simulink model "Model_IPS7"  (R2016a)
settings: Solver=FixedStepAuto  StartTime=0  StopTime=560  FixedStep=1e-5
InitFcn:
  | parametriAM
values from neighbouring files (symbols this model uses):
  Imrn = 7.4    [parametriAM.m]
  Ismax = In*sqrt(2)    [parametriAM.m]
  J = 0.019    [parametriAM.m]    (also in podatki.m = 0.01)
  Ki_Imr = 1000    [parametriAM.m]
  Ki_tok = 5.0    (= 5)    [parametriAM.m]
  Ki_wr = 1000    [parametriAM.m]
  Kp_Imr = 100    [parametriAM.m]
  Kp_tok = 0.05    [parametriAM.m]
  Kp_wr = 50    [parametriAM.m]
  Lm = 0.0493    [parametriAM.m]    (also in podatki.m = 0.2342)
  Lr = 0.05315    [parametriAM.m]    (also in podatki.m = 0.2449)
  Ls = 0.05315    [parametriAM.m]    (also in podatki.m = 0.2449)
  Lst = sigma*Ls    (= 0.00742111947319)    [parametriAM.m]
  naklon = naklon    [parametriAM.m]    (also in staticna_karakteristika.m = 1.0471975512)
  pp = 3    [parametriAM.m]    (also in podatki.m = 2)
  Rs = 0.594    [parametriAM.m]    (also in podatki.m = 3.7)
  sigma = 1 - 1/((1+sigmaR)*(1+sigmaS))    (= 0.13962595434)    [parametriAM.m]
  static_or_dinamic = static_or_dinamic    [parametriAM.m]    (also in potek_toka.m = 0; staticna_karakteristika.m = 5)
  Tr = Lr/Rr    (= 0.0771407837446)    [parametriAM.m]
  Udc = Un*sqrt(2)    [parametriAM.m]
  wb_upper_limit_field_weaking = sqrt((Ls^2+Lst^2)/(2*Lst^2*Ls^2))*Usmax/Ismax    [parametriAM.m]
  wdod = 2000*2*pi/60    (= 209.439510239)    [parametriAM.m]
  wn = Udc/sqrt(Ls^2*(Imrn)^2+Lst^2*(Ismax^2-(Imrn)^2))    [maximalnaelipsa.m]    (also in parametriAM.m = Un/sqrt(Ls^2*(Imrn)^2+Lst^2*(Ismax^2-(Imrn)^2))/pp)
libraries: simulink x25
(part 2 of 2)

== system Model_IPS7/Asinhronski stroj2/napetostni dq model/eq 5.46 ==
  Usd : Inport
  dImr/dt : Inport  Port=2
  Isq : Inport  Port=3
  wmr : Inport  Port=4
  Gain : Gain  Gain=1/(sigma*Ls)
  Gain1 : Gain  Gain=Rs
  Gain2 : Gain  Gain=(1-sigma)*Ls
  Gain3 : Gain  Gain=sigma*Ls
  Integrator : Integrator
  Product : Product  RndMeth=Zero
  Sum : Sum  Inputs=+--+
  Isd : Outport
  wires:
  Gain3/1 -> Sum/4
  Product/1 -> Gain3/1
  Isq/1 -> Product/1
  wmr/1 -> Product/2
  Gain2/1 -> Sum/3
  dImr/dt/1 -> Gain2/1
  Gain1/1 -> Sum/2
  Usd/1 -> Sum/1
  Sum/1 -> Gain/1
  Gain/1 -> Integrator/1
  Integrator/1 -> Gain1/1, Isd/1

== system Model_IPS7/Asinhronski stroj2/napetostni dq model/eq 5.47 ==
  Usq : Inport
  Imr : Inport  Port=2
  Isd : Inport  Port=3
  wmr : Inport  Port=4
  Gain : Gain  Gain=1/(sigma*Ls)
  Gain1 : Gain  Gain=Rs
  Gain2 : Gain  Gain=(1-sigma)*Ls
  Gain3 : Gain  Gain=sigma*Ls
  Integrator : Integrator
  Product : Product  RndMeth=Zero
  Product1 : Product  RndMeth=Zero
  Sum : Sum  Inputs=+---
  Isq : Outport
  wires:
  Gain3/1 -> Sum/4
  Product1/1 -> Gain3/1
  Isd/1 -> Product1/2
  Gain2/1 -> Sum/3
  Product/1 -> Gain2/1
  wmr/1 -> Product1/1, Product/2
  Imr/1 -> Product/1
  Gain1/1 -> Sum/2
  Usq/1 -> Sum/1
  Sum/1 -> Gain/1
  Gain/1 -> Integrator/1
  Integrator/1 -> Gain1/1, Isq/1

== system Model_IPS7/Asinhronski stroj3/Clarke/ABC_ab1 ==
  A : Inport
  B : Inport  Port=2
  C : Inport  Port=3
  Gain1 : Gain  Gain=2
  Gain2 : Gain
  Gain24 : Gain  Gain=sqrt(3)/3
  Sum11 : Sum
  Terminator : Terminator
  alfa : Outport
  beta : Outport  Port=2
  wires:
  A/1 -> Gain2/1, Sum11/1
  Sum11/1 -> Gain24/1
  Gain2/1 -> alfa/1
  Gain24/1 -> beta/1
  B/1 -> Gain1/1
  Gain1/1 -> Sum11/2
  C/1 -> Terminator/1

== system Model_IPS7/Asinhronski stroj3/Inverzni Clarke/ab_ABC ==
  alfa : Inport
  beta : Inport  Port=2
  Gain1 : Gain
  Gain2 : Gain  Gain=-0.5
  Gain25 : Gain  Gain=sqrt(3)/2
  Gain3 : Gain  Gain=sqrt(3)/2
  Gain4 : Gain  Gain=0.5
  Sum10 : Sum
  Sum11 : Sum  Inputs=--
  A : Outport
  B : Outport  Port=2
  C : Outport  Port=3
  wires:
  Sum11/1 -> C/1
  Sum10/1 -> B/1
  Gain1/1 -> A/1
  alfa/1 -> Gain4/1, Gain2/1, Gain1/1
  Gain2/1 -> Sum10/1
  Gain25/1 -> Sum10/2
  Gain4/1 -> Sum11/1
  beta/1 -> Gain3/1, Gain25/1
  Gain3/1 -> Sum11/2

== system Model_IPS7/Asinhronski stroj3/Mehanika/eq 2.19 ==
  M : Inport
  Gain1 : Gain  Gain=1/J
  Integrator : Integrator
  wr : Outport
  wires:
  Gain1/1 -> Integrator/1
  M/1 -> Gain1/1
  Integrator/1 -> wr/1

== system Model_IPS7/Asinhronski stroj3/napetostni dq model/eq 5.35 ==
  Imr : Inport
  Isq : Inport  Port=2
  Gain : Gain  Gain=3*pp/2
  Gain2 : Gain  Gain=Lm*Lm/Lr
  Product : Product  RndMeth=Zero
  Mel : Outport
  wires:
  Imr/1 -> Product/1
  Isq/1 -> Product/2
  Product/1 -> Gain/1
  Gain2/1 -> Mel/1
  Gain/1 -> Gain2/1

== system Model_IPS7/Asinhronski stroj3/napetostni dq model/eq 5.39 ==
  Isd : Inport
  Gain : Gain  Gain=1/Tr
  Integrator : Integrator  InitialCondition=1e-3
  Sum : Sum  Inputs=|+-
  Imr : Outport
  dImr/dt : Outport  Port=2
  wires:
  Isd/1 -> Sum/1
  Integrator/1 -> Imr/1, Sum/2
  Sum/1 -> Gain/1
  Gain/1 -> Integrator/1, dImr/dt/1

== system Model_IPS7/Asinhronski stroj3/napetostni dq model/eq 5.40 ==
  Imr : Inport
  Isq : Inport  Port=2
  wr_el : Inport  Port=3
  Divide : Product  Inputs=*/
  Gain2 : Gain  Gain=Tr
  Saturation : Saturate  UpperLimit=2*pi*50  LowerLimit=-2*pi*50
  Sum : Sum  Inputs=|++
  wmr : Outport
  wires:
  Isq/1 -> Divide/1
  Imr/1 -> Gain2/1
  Gain2/1 -> Divide/2
  Divide/1 -> Saturation/1  "ws"
  wr_el/1 -> Sum/2
  Sum/1 -> wmr/1
  Saturation/1 -> Sum/1

== system Model_IPS7/Asinhronski stroj3/napetostni dq model/eq 5.46 ==
  Usd : Inport
  dImr/dt : Inport  Port=2
  Isq : Inport  Port=3
  wmr : Inport  Port=4
  Gain : Gain  Gain=1/(sigma*Ls)
  Gain1 : Gain  Gain=Rs
  Gain2 : Gain  Gain=(1-sigma)*Ls
  Gain3 : Gain  Gain=sigma*Ls
  Integrator : Integrator
  Product : Product  RndMeth=Zero
  Sum : Sum  Inputs=+--+
  Isd : Outport
  wires:
  Integrator/1 -> Isd/1, Gain1/1
  Gain/1 -> Integrator/1
  Sum/1 -> Gain/1
  Usd/1 -> Sum/1
  Gain1/1 -> Sum/2
  dImr/dt/1 -> Gain2/1
  Gain2/1 -> Sum/3
  wmr/1 -> Product/2
  Isq/1 -> Product/1
  Product/1 -> Gain3/1
  Gain3/1 -> Sum/4

== system Model_IPS7/Asinhronski stroj3/napetostni dq model/eq 5.47 ==
  Usq : Inport
  Imr : Inport  Port=2
  Isd : Inport  Port=3
  wmr : Inport  Port=4
  Gain : Gain  Gain=1/(sigma*Ls)
  Gain1 : Gain  Gain=Rs
  Gain2 : Gain  Gain=(1-sigma)*Ls
  Gain3 : Gain  Gain=sigma*Ls
  Integrator : Integrator
  Product : Product  RndMeth=Zero
  Product1 : Product  RndMeth=Zero
  Sum : Sum  Inputs=+---
  Isq : Outport
  wires:
  Integrator/1 -> Isq/1, Gain1/1
  Gain/1 -> Integrator/1
  Sum/1 -> Gain/1
  Usq/1 -> Sum/1
  Gain1/1 -> Sum/2
  Imr/1 -> Product/1
  wmr/1 -> Product/2, Product1/1
  Product/1 -> Gain2/1
  Gain2/1 -> Sum/3
  Isd/1 -> Product1/2
  Product1/1 -> Gain3/1
  Gain3/1 -> Sum/4

== system Model_IPS7/Regulacija1/Regulacija navora/Limita q toka ==
  Iddej : Inport
  wmr : Inport  Port=2
  Iq* : Inport  Port=3
  0 : Constant  Value=0
  Saturation napetost : simulink/Discontinuities/Saturation Dynamic  OutMin=[]  OutMax=[]  OutDataTypeStr=Inherit: Same as second input  OutDataType=fixdt(1, 16)  OutScaling=2^-10  DoSatur=off
  Saturation presek : simulink/Discontinuities/Saturation Dynamic  OutMin=[]  OutMax=[]  OutDataTypeStr=Inherit: Same as second input  OutDataType=fixdt(1, 16)  OutScaling=2^-10  DoSatur=off
  Saturation tok : simulink/Discontinuities/Saturation Dynamic  OutMin=[]  OutMax=[]  OutDataTypeStr=Inherit: Same as second input  OutDataType=fixdt(1, 16)  OutScaling=2^-10  DoSatur=off
  napetostna limita : Subsystem
  tokovna : Subsystem
  Iqmaxlim : Outport
  Iq*_lim : Outport  Port=2
  wires:
  wmr/1 -> napetostna limita/2(w)
  napetostna limita/1(high) -> Saturation napetost/1, Saturation presek/1
  Iddej/1 -> napetostna limita/1(Iddej), tokovna/1(Id)
  tokovna/2(low) -> Saturation tok/3
  tokovna/1(high) -> Saturation tok/1, Saturation presek/2
  Saturation presek/1 -> Iqmaxlim/1
  Saturation tok/1 -> Saturation napetost/2
  Iq*/1 -> Saturation tok/2
  0/1 -> Saturation presek/3
  napetostna limita/2(low) -> Saturation napetost/3
  Saturation napetost/1 -> Iq*_lim/1

== system Model_IPS7/Regulacija1/Regulacija navora/izracun w_mr ==
  Id : Inport
  Iq : Inport  Port=2
  w : Inport  Port=3
  Constant : Constant  Value=0.00001
  Divide : Product  Inputs=/*
  Gain2 : Gain  Gain=Tr
  Saturation1 : Saturate  UpperLimit=2*pi*50  LowerLimit=-2*pi*50
  Sum : Sum  Inputs=|++
  Sum1 : Sum  Inputs=++|
  Transfer Fcn : TransferFcn  Denominator=[Tr 1]
  wmr : Outport
  wires:
  w/1 -> Sum/2
  Id/1 -> Transfer Fcn/1
  Saturation1/1 -> Sum/1
  Sum/1 -> wmr/1
  Iq/1 -> Divide/2
  Transfer Fcn/1 -> Gain2/1
  Divide/1 -> Saturation1/1
  Gain2/1 -> Sum1/2
  Sum1/1 -> Divide/1
  Constant/1 -> Sum1/1

== system Model_IPS7/Regulacija1/Tok regulator/Dregulator ==
  Id* : Inport
  Iddej : Inport  Port=2
  1/Ti : Gain  Gain=Ki_tok  SaturateOnIntegerOverflow=on  OutDataTypeStr=Inherit: Same as input  ParamDataTypeStr=Inherit: Same as input
  Abs : Abs  ZeroCross=off
  Add2 : Sum  Inputs=+-
  Compare To Zero : simulink/Logic and Bit Operations/Compare To Zero  relop=<=  OutDataTypeStr=boolean  ZeroCross=off
  Integrator : Integrator
  Kp : Gain  Gain=Kp_tok  SaturateOnIntegerOverflow=on  OutDataTypeStr=Inherit: Same as input  ParamDataTypeStr=Inherit: Same as input
  Product : Product
  Saturation : Saturate  UpperLimit=0.990  LowerLimit=-0.990  ZeroCross=off
  Sum1 : Sum  Inputs=|+-
  Sum2 : Sum  Inputs=|++
  Ud*(-1:1) : Outport
  wires:
  Sum1/1 -> Product/1, Kp/1
  Add2/1 -> Abs/1
  Abs/1 -> Compare To Zero/1
  Iddej/1 -> Sum1/2
  1/Ti/1 -> Integrator/1
  Product/1 -> 1/Ti/1
  Kp/1 -> Sum2/1
  Compare To Zero/1 -> Product/2
  Sum2/1 -> Add2/1, Saturation/1
  Integrator/1 -> Sum2/2
  Id*/1 -> Sum1/1
  Saturation/1 -> Add2/2, Ud*(-1:1)/1

== system Model_IPS7/Regulacija1/Tok regulator/Limita Uq ==
  Ud : Inport
  Uq : Inport  Port=2
  Abs : Abs
  Add : Sum  Inputs=+-
  Constant1 : Constant
  Gain : Gain  Gain=-1
  Product3 : Product
  Saturation Dynamic : simulink/Discontinuities/Saturation Dynamic  OutMin=[]  OutMax=[]  OutDataTypeStr=Inherit: Same as second input  OutDataType=fixdt(1, 16)  OutScaling=2^-10  DoSatur=on
  Sqrt : Sqrt  SaturateOnIntegerOverflow=on
  Uq_lim : Outport
  wires:
  Ud/1 -> Product3/1, Product3/2
  Uq/1 -> Saturation Dynamic/2
  Saturation Dynamic/1 -> Uq_lim/1
  Constant1/1 -> Add/1
  Gain/1 -> Saturation Dynamic/3
  Product3/1 -> Add/2
  Add/1 -> Sqrt/1
  Sqrt/1 -> Abs/1
  Abs/1 -> Saturation Dynamic/1, Gain/1

== system Model_IPS7/Regulacija1/Tok regulator/Qregulator ==
  Iqdej : Inport
  Iq* : Inport  Port=2
  Uqlim : Inport  Port=3
  1/Ti1 : Gain  Gain=Ki_tok  SaturateOnIntegerOverflow=on  OutDataTypeStr=Inherit: Same as input  ParamDataTypeStr=Inherit: Same as input
  Abs1 : Abs
  Add1 : Sum  Inputs=+-
  Compare To Zero1 : simulink/Logic and Bit Operations/Compare To Zero  relop=<=  OutDataTypeStr=boolean
  Integrator1 : Integrator
  Kp1 : Gain  Gain=Kp_tok  SaturateOnIntegerOverflow=on  OutDataTypeStr=Inherit: Same as input  ParamDataTypeStr=Inherit: Same as input
  Product1 : Product
  Saturation : Saturate  UpperLimit=1  LowerLimit=-1  ZeroCross=off
  Sum3 : Sum  Inputs=|+-
  Sum4 : Sum  Inputs=|++
  Uq*(-1:1) : Outport
  wires:
  Iq*/1 -> Sum3/1
  Kp1/1 -> Sum4/1
  Integrator1/1 -> Sum4/2
  Sum3/1 -> Kp1/1, Product1/1
  Add1/1 -> Abs1/1
  Compare To Zero1/1 -> Product1/2
  Product1/1 -> 1/Ti1/1
  1/Ti1/1 -> Integrator1/1
  Abs1/1 -> Compare To Zero1/1
  Iqdej/1 -> Sum3/2
  Sum4/1 -> Saturation/1, Add1/1
  Uqlim/1 -> Add1/2
  Saturation/1 -> Uq*(-1:1)/1

== system Model_IPS7/Regulacija1/Transformacije/Clarke ==
  I_123 : Inport
  ABC_ab1 : Subsystem
  Demux : Demux  Outputs=3
  Mux : Mux  Inputs=2
  I_ab : Outport
  wires:
  Mux/1 -> I_ab/1
  ABC_ab1/2(beta) -> Mux/2
  ABC_ab1/1(alfa) -> Mux/1
  Demux/3 -> ABC_ab1/3(C)
  Demux/2 -> ABC_ab1/2(B)
  Demux/1 -> ABC_ab1/1(A)
  I_123/1 -> Demux/1

== system Model_IPS7/Regulacija1/Transformacije/Inverzni Clarke ==
  U_ab : Inport
  Demux : Demux  Outputs=2
  Mux : Mux  Inputs=3
  ab_ABC : Subsystem
  U_123 : Outport
  wires:
  ab_ABC/3(C) -> Mux/3
  ab_ABC/2(B) -> Mux/2
  ab_ABC/1(A) -> Mux/1
  Demux/2 -> ab_ABC/2(beta)
  Demux/1 -> ab_ABC/1(alfa)
  U_ab/1 -> Demux/1
  Mux/1 -> U_123/1

== system Model_IPS7/Regulacija1/Transformacije/Inverzni Park ==
  kot : Inport
  U_dq : Inport  Port=2
  Demux : Demux  Outputs=2
  Mux : Mux  Inputs=2
  "Sum1 " : Sum  Inputs=+-  SaturateOnIntegerOverflow=on  InputSameDT=on  OutDataTypeStr=Inherit: Same as first input
  Sum2 : Sum  SaturateOnIntegerOverflow=on  InputSameDT=on  OutDataTypeStr=Inherit: Same as first input
  cos : Fcn  Expr=cos(u)
  sin : Fcn  Expr=sin(u)
  x_d*cos : Product  SaturateOnIntegerOverflow=on  RndMeth=Zero  InputSameDT=on  OutDataTypeStr=Inherit: Same as first input
  x_d*sin : Product  SaturateOnIntegerOverflow=on  RndMeth=Zero  InputSameDT=on  OutDataTypeStr=Inherit: Same as first input
  x_q*cos : Product  SaturateOnIntegerOverflow=on  RndMeth=Zero  InputSameDT=on  OutDataTypeStr=Inherit: Same as first input
  "x_q*sin " : Product  SaturateOnIntegerOverflow=on  RndMeth=Zero  InputSameDT=on  OutDataTypeStr=Inherit: Same as first input
  U_ab : Outport
  wires:
  Mux/1 -> U_ab/1
  U_dq/1 -> Demux/1
  Demux/1 -> x_d*sin/1, x_d*cos/1
  Demux/2 -> "x_q*sin "/1, x_q*cos/1
  cos/1 -> x_q*cos/2, x_d*cos/2
  sin/1 -> "x_q*sin "/2, x_d*sin/2
  x_d*cos/1 -> "Sum1 "/1
  "x_q*sin "/1 -> "Sum1 "/2
  x_q*cos/1 -> Sum2/2
  x_d*sin/1 -> Sum2/1
  "Sum1 "/1 -> Mux/1
  Sum2/1 -> Mux/2
  kot/1 -> cos/1, sin/1

== system Model_IPS7/Regulacija1/Transformacije/Park ==
  I_ab : Inport
  kot : Inport  Port=2
  Demux : Demux  Outputs=2
  Mux : Mux  Inputs=2
  "Sum1 " : Sum  SaturateOnIntegerOverflow=on  InputSameDT=on  OutDataTypeStr=Inherit: Same as first input
  Sum2 : Sum  Inputs=-+  SaturateOnIntegerOverflow=on  InputSameDT=on  OutDataTypeStr=Inherit: Same as first input
  cos : Fcn  Expr=cos(u)
  sin : Fcn  Expr=sin(u)
  x_a*cos : Product  SaturateOnIntegerOverflow=on  RndMeth=Zero  InputSameDT=on  OutDataTypeStr=Inherit: Same as first input
  x_a*sin : Product  SaturateOnIntegerOverflow=on  RndMeth=Zero  InputSameDT=on  OutDataTypeStr=Inherit: Same as first input
  x_b*cos : Product  SaturateOnIntegerOverflow=on  RndMeth=Zero  InputSameDT=on  OutDataTypeStr=Inherit: Same as first input
  "x_b*sin " : Product  SaturateOnIntegerOverflow=on  RndMeth=Zero  InputSameDT=on  OutDataTypeStr=Inherit: Same as first input
  I_dq : Outport
  wires:
  Mux/1 -> I_dq/1
  I_ab/1 -> Demux/1
  Demux/1 -> x_a*sin/1, x_a*cos/1
  Demux/2 -> "x_b*sin "/1, x_b*cos/1
  cos/1 -> x_b*cos/2, x_a*cos/2
  sin/1 -> "x_b*sin "/2, x_a*sin/2
  x_a*cos/1 -> "Sum1 "/1
  "x_b*sin "/1 -> "Sum1 "/2
  x_b*cos/1 -> Sum2/2
  x_a*sin/1 -> Sum2/1
  "Sum1 "/1 -> Mux/1
  Sum2/1 -> Mux/2
  kot/1 -> cos/1, sin/1

== system Model_IPS7/Regulacija2/Regulacija navora/Limita q toka ==
  Iddej : Inport
  wfdb : Inport  Port=2
  Iq* : Inport  Port=3
  0 : Constant  Value=0
  Saturation napetost : simulink/Discontinuities/Saturation Dynamic  OutMin=[]  OutMax=[]  OutDataTypeStr=Inherit: Same as second input  OutDataType=fixdt(1, 16)  OutScaling=2^-10  DoSatur=off
  Saturation presek : simulink/Discontinuities/Saturation Dynamic  OutMin=[]  OutMax=[]  OutDataTypeStr=Inherit: Same as second input  OutDataType=fixdt(1, 16)  OutScaling=2^-10  DoSatur=off
  Saturation tok : simulink/Discontinuities/Saturation Dynamic  OutMin=[]  OutMax=[]  OutDataTypeStr=Inherit: Same as second input  OutDataType=fixdt(1, 16)  OutScaling=2^-10  DoSatur=off
  napetostna limita : Subsystem
  tokovna : Subsystem
  Iqmaxlim : Outport
  Iq*_lim : Outport  Port=2
  wires:
  wfdb/1 -> napetostna limita/2(w)
  napetostna limita/1(high) -> Saturation napetost/1, Saturation presek/1
  Iddej/1 -> napetostna limita/1(Iddej), tokovna/1(Id)
  tokovna/2(low) -> Saturation tok/3
  tokovna/1(high) -> Saturation tok/1, Saturation presek/2
  Saturation presek/1 -> Iqmaxlim/1
  Saturation tok/1 -> Saturation napetost/2
  Iq*/1 -> Saturation tok/2
  0/1 -> Saturation presek/3
  Saturation napetost/1 -> Iq*_lim/1
  napetostna limita/2(low) -> Saturation napetost/3

== system Model_IPS7/Regulacija2/Regulacija navora/izracun w_mr ==
  Id : Inport
  Iq : Inport  Port=2
  w : Inport  Port=3
  Constant : Constant  Value=0.00001
  Divide : Product  Inputs=/*
  Gain2 : Gain  Gain=Tr
  Saturation1 : Saturate  UpperLimit=2*pi*50  LowerLimit=-2*pi*50
  Sum : Sum  Inputs=|++
  Sum1 : Sum  Inputs=++|
  Transfer Fcn : TransferFcn  Denominator=[Tr 1]
  wmr : Outport
  wires:
  w/1 -> Sum/2
  Id/1 -> Transfer Fcn/1
  Saturation1/1 -> Sum/1
  Sum/1 -> wmr/1
  Iq/1 -> Divide/2
  Transfer Fcn/1 -> Gain2/1
  Divide/1 -> Saturation1/1
  Gain2/1 -> Sum1/2
  Sum1/1 -> Divide/1
  Constant/1 -> Sum1/1

== system Model_IPS7/Regulacija2/Tok regulator/Dregulator ==
  Id* : Inport
  Iddej : Inport  Port=2
  1/Ti : Gain  Gain=Ki_tok  SaturateOnIntegerOverflow=on  OutDataTypeStr=Inherit: Same as input  ParamDataTypeStr=Inherit: Same as input
  Abs : Abs  ZeroCross=off
  Add2 : Sum  Inputs=+-
  Compare To Zero : simulink/Logic and Bit Operations/Compare To Zero  relop=<=  OutDataTypeStr=boolean  ZeroCross=off
  Integrator : Integrator
  Kp : Gain  Gain=Kp_tok  SaturateOnIntegerOverflow=on  OutDataTypeStr=Inherit: Same as input  ParamDataTypeStr=Inherit: Same as input
  Product : Product
  Saturation : Saturate  UpperLimit=0.990  LowerLimit=-0.990  ZeroCross=off
  Sum1 : Sum  Inputs=|+-
  Sum2 : Sum  Inputs=|++
  Ud*(-1:1) : Outport
  wires:
  Sum1/1 -> Product/1, Kp/1
  Add2/1 -> Abs/1
  Abs/1 -> Compare To Zero/1
  Iddej/1 -> Sum1/2
  1/Ti/1 -> Integrator/1
  Product/1 -> 1/Ti/1
  Kp/1 -> Sum2/1
  Compare To Zero/1 -> Product/2
  Sum2/1 -> Add2/1, Saturation/1
  Integrator/1 -> Sum2/2
  Id*/1 -> Sum1/1
  Saturation/1 -> Add2/2, Ud*(-1:1)/1

== system Model_IPS7/Regulacija2/Tok regulator/Limita Uq ==
  Ud : Inport
  Uq : Inport  Port=2
  Abs : Abs
  Add : Sum  Inputs=+-
  Constant1 : Constant
  Gain : Gain  Gain=-1
  Product3 : Product
  Saturation Dynamic : simulink/Discontinuities/Saturation Dynamic  OutMin=[]  OutMax=[]  OutDataTypeStr=Inherit: Same as second input  OutDataType=fixdt(1, 16)  OutScaling=2^-10  DoSatur=off
  Sqrt : Sqrt  SaturateOnIntegerOverflow=on
  Uq_lim : Outport
  wires:
  Ud/1 -> Product3/1, Product3/2
  Uq/1 -> Saturation Dynamic/2
  Saturation Dynamic/1 -> Uq_lim/1
  Constant1/1 -> Add/1
  Gain/1 -> Saturation Dynamic/3
  Product3/1 -> Add/2
  Add/1 -> Sqrt/1
  Sqrt/1 -> Abs/1
  Abs/1 -> Saturation Dynamic/1, Gain/1

== system Model_IPS7/Regulacija2/Tok regulator/Qregulator ==
  Iqdej : Inport
  Iq* : Inport  Port=2
  Uqlim : Inport  Port=3
  1/Ti1 : Gain  Gain=Ki_tok  SaturateOnIntegerOverflow=on  OutDataTypeStr=Inherit: Same as input  ParamDataTypeStr=Inherit: Same as input
  Abs1 : Abs
  Add1 : Sum  Inputs=+-
  Compare To Zero1 : simulink/Logic and Bit Operations/Compare To Zero  relop=<=  OutDataTypeStr=boolean
  Integrator1 : Integrator
  Kp1 : Gain  Gain=Kp_tok  SaturateOnIntegerOverflow=on  OutDataTypeStr=Inherit: Same as input  ParamDataTypeStr=Inherit: Same as input
  Product1 : Product
  Sum3 : Sum  Inputs=|+-
  Sum4 : Sum  Inputs=|++
  Uq*(-1:1) : Outport
  wires:
  Iq*/1 -> Sum3/1
  Kp1/1 -> Sum4/1
  Integrator1/1 -> Sum4/2
  Sum3/1 -> Kp1/1, Product1/1
  Add1/1 -> Abs1/1
  Compare To Zero1/1 -> Product1/2
  Product1/1 -> 1/Ti1/1
  1/Ti1/1 -> Integrator1/1
  Abs1/1 -> Compare To Zero1/1
  Iqdej/1 -> Sum3/2
  Sum4/1 -> Uq*(-1:1)/1, Add1/1
  Uqlim/1 -> Add1/2

== system Model_IPS7/Regulacija2/Transformacije/Clarke ==
  I_123 : Inport
  ABC_ab1 : Subsystem
  Demux : Demux  Outputs=3
  Mux : Mux  Inputs=2
  I_ab : Outport
  wires:
  Mux/1 -> I_ab/1
  ABC_ab1/2(beta) -> Mux/2
  ABC_ab1/1(alfa) -> Mux/1
  Demux/3 -> ABC_ab1/3(C)
  Demux/2 -> ABC_ab1/2(B)
  Demux/1 -> ABC_ab1/1(A)
  I_123/1 -> Demux/1

== system Model_IPS7/Regulacija2/Transformacije/Inverzni Clarke ==
  U_ab : Inport
  Demux : Demux  Outputs=2
  Mux : Mux  Inputs=3
  ab_ABC : Subsystem
  U_123 : Outport
  wires:
  ab_ABC/3(C) -> Mux/3
  ab_ABC/2(B) -> Mux/2
  ab_ABC/1(A) -> Mux/1
  Demux/2 -> ab_ABC/2(beta)
  Demux/1 -> ab_ABC/1(alfa)
  U_ab/1 -> Demux/1
  Mux/1 -> U_123/1

== system Model_IPS7/Regulacija2/Transformacije/Inverzni Park ==
  kot : Inport
  U_dq : Inport  Port=2
  Demux : Demux  Outputs=2
  Mux : Mux  Inputs=2
  "Sum1 " : Sum  Inputs=+-  SaturateOnIntegerOverflow=on  InputSameDT=on  OutDataTypeStr=Inherit: Same as first input
  Sum2 : Sum  SaturateOnIntegerOverflow=on  InputSameDT=on  OutDataTypeStr=Inherit: Same as first input
  cos : Fcn  Expr=cos(u)
  sin : Fcn  Expr=sin(u)
  x_d*cos : Product  SaturateOnIntegerOverflow=on  RndMeth=Zero  InputSameDT=on  OutDataTypeStr=Inherit: Same as first input
  x_d*sin : Product  SaturateOnIntegerOverflow=on  RndMeth=Zero  InputSameDT=on  OutDataTypeStr=Inherit: Same as first input
  x_q*cos : Product  SaturateOnIntegerOverflow=on  RndMeth=Zero  InputSameDT=on  OutDataTypeStr=Inherit: Same as first input
  "x_q*sin " : Product  SaturateOnIntegerOverflow=on  RndMeth=Zero  InputSameDT=on  OutDataTypeStr=Inherit: Same as first input
  U_ab : Outport
  wires:
  Mux/1 -> U_ab/1
  U_dq/1 -> Demux/1
  Demux/1 -> x_d*sin/1, x_d*cos/1
  Demux/2 -> "x_q*sin "/1, x_q*cos/1
  cos/1 -> x_q*cos/2, x_d*cos/2
  sin/1 -> "x_q*sin "/2, x_d*sin/2
  x_d*cos/1 -> "Sum1 "/1
  "x_q*sin "/1 -> "Sum1 "/2
  x_q*cos/1 -> Sum2/2
  x_d*sin/1 -> Sum2/1
  "Sum1 "/1 -> Mux/1
  Sum2/1 -> Mux/2
  kot/1 -> cos/1, sin/1

== system Model_IPS7/Regulacija2/Transformacije/Park ==
  I_ab : Inport
  kot : Inport  Port=2
  Demux : Demux  Outputs=2
  Mux : Mux  Inputs=2
  "Sum1 " : Sum  SaturateOnIntegerOverflow=on  InputSameDT=on  OutDataTypeStr=Inherit: Same as first input
  Sum2 : Sum  Inputs=-+  SaturateOnIntegerOverflow=on  InputSameDT=on  OutDataTypeStr=Inherit: Same as first input
  cos : Fcn  Expr=cos(u)
  sin : Fcn  Expr=sin(u)
  x_a*cos : Product  SaturateOnIntegerOverflow=on  RndMeth=Zero  InputSameDT=on  OutDataTypeStr=Inherit: Same as first input
  x_a*sin : Product  SaturateOnIntegerOverflow=on  RndMeth=Zero  InputSameDT=on  OutDataTypeStr=Inherit: Same as first input
  x_b*cos : Product  SaturateOnIntegerOverflow=on  RndMeth=Zero  InputSameDT=on  OutDataTypeStr=Inherit: Same as first input
  "x_b*sin " : Product  SaturateOnIntegerOverflow=on  RndMeth=Zero  InputSameDT=on  OutDataTypeStr=Inherit: Same as first input
  I_dq : Outport
  wires:
  Mux/1 -> I_dq/1
  I_ab/1 -> Demux/1
  Demux/1 -> x_a*sin/1, x_a*cos/1
  Demux/2 -> "x_b*sin "/1, x_b*cos/1
  cos/1 -> x_b*cos/2, x_a*cos/2
  sin/1 -> "x_b*sin "/2, x_a*sin/2
  x_a*cos/1 -> "Sum1 "/1
  "x_b*sin "/1 -> "Sum1 "/2
  x_b*cos/1 -> Sum2/2
  x_a*sin/1 -> Sum2/1
  "Sum1 "/1 -> Mux/1
  Sum2/1 -> Mux/2
  kot/1 -> cos/1, sin/1

== system Model_IPS7/Regulacija3/Regulacija navora/Limita q toka ==
  Iddej : Inport
  wfdb : Inport  Port=2
  Iq* : Inport  Port=3
  0 : Constant  Value=0
  Saturation presek : simulink/Discontinuities/Saturation Dynamic  OutMin=[]  OutMax=[]  OutDataTypeStr=Inherit: Same as second input  OutDataType=fixdt(1, 16)  OutScaling=2^-10  DoSatur=off
  Saturation tok : simulink/Discontinuities/Saturation Dynamic  OutMin=[]  OutMax=[]  OutDataTypeStr=Inherit: Same as second input  OutDataType=fixdt(1, 16)  OutScaling=2^-10  DoSatur=off
  napetostna limita : Subsystem
  tokovna : Subsystem
  Iqmaxlim : Outport
  Iq*_lim : Outport  Port=2
  wires:
  0/1 -> Saturation presek/3
  Iq*/1 -> Saturation tok/2
  Saturation tok/1 -> Iq*_lim/1
  Saturation presek/1 -> Iqmaxlim/1
  tokovna/1(high) -> Saturation presek/2, Saturation tok/1
  tokovna/2(low) -> Saturation tok/3
  Iddej/1 -> tokovna/1(Id), napetostna limita/1(Iddej)
  napetostna limita/1(high) -> Saturation presek/1
  wfdb/1 -> napetostna limita/2(w)

== system Model_IPS7/Regulacija3/Regulacija navora/izracun w_mr ==
  Id : Inport
  Iq : Inport  Port=2
  w : Inport  Port=3
  Constant : Constant  Value=0.00001
  Divide : Product  Inputs=/*
  Gain2 : Gain  Gain=Tr
  Saturation1 : Saturate  UpperLimit=2*pi*50  LowerLimit=-2*pi*50
  Sum : Sum  Inputs=|++
  Sum1 : Sum  Inputs=++|
  Transfer Fcn : TransferFcn  Denominator=[Tr 1]
  wmr : Outport
  wires:
  Constant/1 -> Sum1/1
  Sum1/1 -> Divide/1
  Gain2/1 -> Sum1/2
  Divide/1 -> Saturation1/1
  Transfer Fcn/1 -> Gain2/1
  Iq/1 -> Divide/2
  Sum/1 -> wmr/1
  Saturation1/1 -> Sum/1
  Id/1 -> Transfer Fcn/1
  w/1 -> Sum/2

== system Model_IPS7/Regulacija3/Tok regulator/Dregulator ==
  Id* : Inport
  Iddej : Inport  Port=2
  1/Ti : Gain  Gain=Ki_tok  SaturateOnIntegerOverflow=on  OutDataTypeStr=Inherit: Same as input  ParamDataTypeStr=Inherit: Same as input
  Abs : Abs  ZeroCross=off
  Add2 : Sum  Inputs=+-
  Compare To Zero : simulink/Logic and Bit Operations/Compare To Zero  relop=<=  OutDataTypeStr=boolean  ZeroCross=off
  Integrator : Integrator
  Kp : Gain  Gain=Kp_tok  SaturateOnIntegerOverflow=on  OutDataTypeStr=Inherit: Same as input  ParamDataTypeStr=Inherit: Same as input
  Product : Product
  Saturation : Saturate  UpperLimit=0.990  LowerLimit=-0.990  ZeroCross=off
  Sum1 : Sum  Inputs=|+-
  Sum2 : Sum  Inputs=|++
  Ud*(-1:1) : Outport
  wires:
  Saturation/1 -> Ud*(-1:1)/1, Add2/2
  Id*/1 -> Sum1/1
  Integrator/1 -> Sum2/2
  Sum2/1 -> Saturation/1, Add2/1
  Compare To Zero/1 -> Product/2
  Kp/1 -> Sum2/1
  Product/1 -> 1/Ti/1
  1/Ti/1 -> Integrator/1
  Iddej/1 -> Sum1/2
  Abs/1 -> Compare To Zero/1
  Add2/1 -> Abs/1
  Sum1/1 -> Kp/1, Product/1

== system Model_IPS7/Regulacija3/Tok regulator/Limita Uq ==
  Ud : Inport
  Uq : Inport  Port=2
  Abs : Abs
  Add : Sum  Inputs=+-
  Constant1 : Constant
  Gain : Gain  Gain=-1
  Product3 : Product
  Saturation Dynamic : simulink/Discontinuities/Saturation Dynamic  OutMin=[]  OutMax=[]  OutDataTypeStr=Inherit: Same as second input  OutDataType=fixdt(1, 16)  OutScaling=2^-10  DoSatur=off
  Sqrt : Sqrt  SaturateOnIntegerOverflow=on
  Uq_lim : Outport
  wires:
  Abs/1 -> Gain/1, Saturation Dynamic/1
  Sqrt/1 -> Abs/1
  Add/1 -> Sqrt/1
  Product3/1 -> Add/2
  Gain/1 -> Saturation Dynamic/3
  Constant1/1 -> Add/1
  Saturation Dynamic/1 -> Uq_lim/1
  Uq/1 -> Saturation Dynamic/2
  Ud/1 -> Product3/2, Product3/1

== system Model_IPS7/Regulacija3/Tok regulator/Qregulator ==
  Iqdej : Inport
  Iq* : Inport  Port=2
  Uqlim : Inport  Port=3
  1/Ti1 : Gain  Gain=Ki_tok  SaturateOnIntegerOverflow=on  OutDataTypeStr=Inherit: Same as input  ParamDataTypeStr=Inherit: Same as input
  Abs1 : Abs
  Add1 : Sum  Inputs=+-
  Compare To Zero1 : simulink/Logic and Bit Operations/Compare To Zero  relop=<=  OutDataTypeStr=boolean
  Integrator1 : Integrator
  Kp1 : Gain  Gain=Kp_tok  SaturateOnIntegerOverflow=on  OutDataTypeStr=Inherit: Same as input  ParamDataTypeStr=Inherit: Same as input
  Product1 : Product
  Sum3 : Sum  Inputs=|+-
  Sum4 : Sum  Inputs=|++
  Uq*(-1:1) : Outport
  wires:
  Uqlim/1 -> Add1/2
  Sum4/1 -> Add1/1, Uq*(-1:1)/1
  Iqdej/1 -> Sum3/2
  Abs1/1 -> Compare To Zero1/1
  1/Ti1/1 -> Integrator1/1
  Product1/1 -> 1/Ti1/1
  Compare To Zero1/1 -> Product1/2
  Add1/1 -> Abs1/1
  Sum3/1 -> Product1/1, Kp1/1
  Integrator1/1 -> Sum4/2
  Kp1/1 -> Sum4/1
  Iq*/1 -> Sum3/1

== system Model_IPS7/Regulacija3/Transformacije/Clarke ==
  I_123 : Inport
  ABC_ab1 : Subsystem
  Demux : Demux  Outputs=3
  Mux : Mux  Inputs=2
  I_ab : Outport
  wires:
  I_123/1 -> Demux/1
  Demux/1 -> ABC_ab1/1(A)
  Demux/2 -> ABC_ab1/2(B)
  Demux/3 -> ABC_ab1/3(C)
  ABC_ab1/1(alfa) -> Mux/1
  ABC_ab1/2(beta) -> Mux/2
  Mux/1 -> I_ab/1

== system Model_IPS7/Regulacija3/Transformacije/Inverzni Clarke ==
  U_ab : Inport
  Demux : Demux  Outputs=2
  Mux : Mux  Inputs=3
  ab_ABC : Subsystem
  U_123 : Outport
  wires:
  Mux/1 -> U_123/1
  U_ab/1 -> Demux/1
  Demux/1 -> ab_ABC/1(alfa)
  Demux/2 -> ab_ABC/2(beta)
  ab_ABC/1(A) -> Mux/1
  ab_ABC/2(B) -> Mux/2
  ab_ABC/3(C) -> Mux/3

== system Model_IPS7/Regulacija3/Transformacije/Inverzni Park ==
  kot : Inport
  U_dq : Inport  Port=2
  Demux : Demux  Outputs=2
  Mux : Mux  Inputs=2
  "Sum1 " : Sum  Inputs=+-  SaturateOnIntegerOverflow=on  InputSameDT=on  OutDataTypeStr=Inherit: Same as first input
  Sum2 : Sum  SaturateOnIntegerOverflow=on  InputSameDT=on  OutDataTypeStr=Inherit: Same as first input
  cos : Fcn  Expr=cos(u)
  sin : Fcn  Expr=sin(u)
  x_d*cos : Product  SaturateOnIntegerOverflow=on  RndMeth=Zero  InputSameDT=on  OutDataTypeStr=Inherit: Same as first input
  x_d*sin : Product  SaturateOnIntegerOverflow=on  RndMeth=Zero  InputSameDT=on  OutDataTypeStr=Inherit: Same as first input
  x_q*cos : Product  SaturateOnIntegerOverflow=on  RndMeth=Zero  InputSameDT=on  OutDataTypeStr=Inherit: Same as first input
  "x_q*sin " : Product  SaturateOnIntegerOverflow=on  RndMeth=Zero  InputSameDT=on  OutDataTypeStr=Inherit: Same as first input
  U_ab : Outport
  wires:
  kot/1 -> sin/1, cos/1
  Sum2/1 -> Mux/2
  "Sum1 "/1 -> Mux/1
  x_d*sin/1 -> Sum2/1
  x_q*cos/1 -> Sum2/2
  "x_q*sin "/1 -> "Sum1 "/2
  x_d*cos/1 -> "Sum1 "/1
  sin/1 -> x_d*sin/2, "x_q*sin "/2
  cos/1 -> x_d*cos/2, x_q*cos/2
  Demux/2 -> x_q*cos/1, "x_q*sin "/1
  Demux/1 -> x_d*cos/1, x_d*sin/1
  U_dq/1 -> Demux/1
  Mux/1 -> U_ab/1

== system Model_IPS7/Regulacija3/Transformacije/Park ==
  I_ab : Inport
  kot : Inport  Port=2
  Demux : Demux  Outputs=2
  Mux : Mux  Inputs=2
  "Sum1 " : Sum  SaturateOnIntegerOverflow=on  InputSameDT=on  OutDataTypeStr=Inherit: Same as first input
  Sum2 : Sum  Inputs=-+  SaturateOnIntegerOverflow=on  InputSameDT=on  OutDataTypeStr=Inherit: Same as first input
  cos : Fcn  Expr=cos(u)
  sin : Fcn  Expr=sin(u)
  x_a*cos : Product  SaturateOnIntegerOverflow=on  RndMeth=Zero  InputSameDT=on  OutDataTypeStr=Inherit: Same as first input
  x_a*sin : Product  SaturateOnIntegerOverflow=on  RndMeth=Zero  InputSameDT=on  OutDataTypeStr=Inherit: Same as first input
  x_b*cos : Product  SaturateOnIntegerOverflow=on  RndMeth=Zero  InputSameDT=on  OutDataTypeStr=Inherit: Same as first input
  "x_b*sin " : Product  SaturateOnIntegerOverflow=on  RndMeth=Zero  InputSameDT=on  OutDataTypeStr=Inherit: Same as first input
  I_dq : Outport
  wires:
  kot/1 -> sin/1, cos/1
  Sum2/1 -> Mux/2
  "Sum1 "/1 -> Mux/1
  x_a*sin/1 -> Sum2/1
  x_b*cos/1 -> Sum2/2
  "x_b*sin "/1 -> "Sum1 "/2
  x_a*cos/1 -> "Sum1 "/1
  sin/1 -> x_a*sin/2, "x_b*sin "/2
  cos/1 -> x_a*cos/2, x_b*cos/2
  Demux/2 -> x_b*cos/1, "x_b*sin "/1
  Demux/1 -> x_a*cos/1, x_a*sin/1
  I_ab/1 -> Demux/1
  Mux/1 -> I_dq/1

== system Model_IPS7/Regulacija1/Regulacija navora/Limita q toka/napetostna limita ==
  Iddej : Inport
  w : Inport  Port=2
  Abs : Abs
  Abs1 : Abs
  Add1 : Sum  Inputs=-+
  Constant : Constant
  Divide : Product  Inputs=*/
  Gain : Gain  Gain=-1
  Product2 : Product
  Product3 : Product
  Saturation : Saturate  UpperLimit=1  LowerLimit=0
  Sqrt : Sqrt  SaturateOnIntegerOverflow=on
  a : Subsystem
  b : Subsystem
  high : Outport
  low : Outport  Port=2
  wires:
  Sqrt/1 -> Product3/1
  Iddej/1 -> Divide/1
  Divide/1 -> Product2/1, Product2/2
  Constant/1 -> Add1/2
  w/1 -> Abs1/1
  Product3/1 -> Abs/1
  Add1/1 -> Sqrt/1
  b/1(b) -> Product3/2
  Gain/1 -> low/1
  a/1(a) -> Divide/2
  Abs/1 -> high/1, Gain/1
  Abs1/1 -> b/1(w), a/1(w)
  Product2/1 -> Saturation/1
  Saturation/1 -> Add1/1

== system Model_IPS7/Regulacija1/Regulacija navora/Limita q toka/tokovna ==
  Id : Inport
  Abs : Abs
  Constant : Constant  Value=Ismax^2
  Gain2 : Gain  Gain=-1
  Product1 : Product
  Saturation : Saturate  UpperLimit=Ismax^2  LowerLimit=0
  Sqrt : Sqrt  SaturateOnIntegerOverflow=on
  Subtract : Sum  Inputs=+-
  high : Outport
  low : Outport  Port=2
  wires:
  Sqrt/1 -> Abs/1
  Id/1 -> Product1/2, Product1/1
  Gain2/1 -> low/1
  Constant/1 -> Subtract/1
  Product1/1 -> Subtract/2
  Abs/1 -> high/1, Gain2/1
  Subtract/1 -> Saturation/1
  Saturation/1 -> Sqrt/1

== system Model_IPS7/Regulacija1/Transformacije/Clarke/ABC_ab1 ==
  A : Inport
  B : Inport  Port=2
  C : Inport  Port=3
  Gain1 : Gain  Gain=2
  Gain2 : Gain
  Gain24 : Gain  Gain=sqrt(3)/3
  Sum11 : Sum
  Terminator : Terminator
  alfa : Outport
  beta : Outport  Port=2
  wires:
  C/1 -> Terminator/1
  Gain1/1 -> Sum11/2
  B/1 -> Gain1/1
  Gain24/1 -> beta/1
  Gain2/1 -> alfa/1
  Sum11/1 -> Gain24/1
  A/1 -> Sum11/1, Gain2/1

== system Model_IPS7/Regulacija1/Transformacije/Inverzni Clarke/ab_ABC ==
  alfa : Inport
  beta : Inport  Port=2
  Gain1 : Gain
  Gain2 : Gain  Gain=-0.5
  Gain25 : Gain  Gain=sqrt(3)/2
  Gain3 : Gain  Gain=sqrt(3)/2
  Gain4 : Gain  Gain=0.5
  Sum10 : Sum
  Sum11 : Sum  Inputs=--
  A : Outport
  B : Outport  Port=2
  C : Outport  Port=3
  wires:
  Gain3/1 -> Sum11/2
  beta/1 -> Gain25/1, Gain3/1
  Gain4/1 -> Sum11/1
  Gain25/1 -> Sum10/2
  Gain2/1 -> Sum10/1
  alfa/1 -> Gain1/1, Gain2/1, Gain4/1
  Gain1/1 -> A/1
  Sum10/1 -> B/1
  Sum11/1 -> C/1

== system Model_IPS7/Regulacija2/Regulacija navora/Limita q toka/napetostna limita ==
  Iddej : Inport
  w : Inport  Port=2
  Abs : Abs
  Abs1 : Abs
  Add1 : Sum  Inputs=-+
  Constant : Constant
  Divide : Product  Inputs=*/
  Gain : Gain  Gain=-1
  Product2 : Product
  Product3 : Product
  Saturation : Saturate  UpperLimit=1  LowerLimit=0
  Sqrt : Sqrt  SaturateOnIntegerOverflow=on
  a : Subsystem
  b : Subsystem
  high : Outport
  low : Outport  Port=2
  wires:
  Sqrt/1 -> Product3/1
  Iddej/1 -> Divide/1
  Divide/1 -> Product2/1, Product2/2
  Constant/1 -> Add1/2
  w/1 -> Abs1/1
  Product3/1 -> Abs/1
  Add1/1 -> Sqrt/1
  b/1(b) -> Product3/2
  Gain/1 -> low/1
  a/1(a) -> Divide/2
  Abs/1 -> high/1, Gain/1
  Abs1/1 -> b/1(w), a/1(w)
  Product2/1 -> Saturation/1
  Saturation/1 -> Add1/1

== system Model_IPS7/Regulacija2/Regulacija navora/Limita q toka/tokovna ==
  Id : Inport
  Abs : Abs
  Constant : Constant  Value=Ismax^2
  Gain2 : Gain  Gain=-1
  Product1 : Product
  Saturation : Saturate  UpperLimit=Ismax^2  LowerLimit=0
  Sqrt : Sqrt  SaturateOnIntegerOverflow=on
  Subtract : Sum  Inputs=+-
  high : Outport
  low : Outport  Port=2
  wires:
  Sqrt/1 -> Abs/1
  Id/1 -> Product1/2, Product1/1
  Gain2/1 -> low/1
  Constant/1 -> Subtract/1
  Product1/1 -> Subtract/2
  Abs/1 -> high/1, Gain2/1
  Subtract/1 -> Saturation/1
  Saturation/1 -> Sqrt/1

== system Model_IPS7/Regulacija2/Transformacije/Clarke/ABC_ab1 ==
  A : Inport
  B : Inport  Port=2
  C : Inport  Port=3
  Gain1 : Gain  Gain=2
  Gain2 : Gain
  Gain24 : Gain  Gain=sqrt(3)/3
  Sum11 : Sum
  Terminator : Terminator
  alfa : Outport
  beta : Outport  Port=2
  wires:
  C/1 -> Terminator/1
  Gain1/1 -> Sum11/2
  B/1 -> Gain1/1
  Gain24/1 -> beta/1
  Gain2/1 -> alfa/1
  Sum11/1 -> Gain24/1
  A/1 -> Sum11/1, Gain2/1

== system Model_IPS7/Regulacija2/Transformacije/Inverzni Clarke/ab_ABC ==
  alfa : Inport
  beta : Inport  Port=2
  Gain1 : Gain
  Gain2 : Gain  Gain=-0.5
  Gain25 : Gain  Gain=sqrt(3)/2
  Gain3 : Gain  Gain=sqrt(3)/2
  Gain4 : Gain  Gain=0.5
  Sum10 : Sum
  Sum11 : Sum  Inputs=--
  A : Outport
  B : Outport  Port=2
  C : Outport  Port=3
  wires:
  Gain3/1 -> Sum11/2
  beta/1 -> Gain25/1, Gain3/1
  Gain4/1 -> Sum11/1
  Gain25/1 -> Sum10/2
  Gain2/1 -> Sum10/1
  alfa/1 -> Gain1/1, Gain2/1, Gain4/1
  Gain1/1 -> A/1
  Sum10/1 -> B/1
  Sum11/1 -> C/1

== system Model_IPS7/Regulacija3/Regulacija navora/Limita q toka/napetostna limita ==
  Iddej : Inport
  w : Inport  Port=2
  Abs : Abs
  Abs1 : Abs
  Add1 : Sum  Inputs=-+
  Constant : Constant
  Divide : Product  Inputs=*/
  Product2 : Product
  Product3 : Product
  Saturation : Saturate  UpperLimit=1  LowerLimit=0
  Sqrt : Sqrt  SaturateOnIntegerOverflow=on
  a : Subsystem
  b : Subsystem
  high : Outport
  wires:
  Saturation/1 -> Add1/1
  Product2/1 -> Saturation/1
  Abs1/1 -> a/1(w), b/1(w)
  Abs/1 -> high/1
  a/1(a) -> Divide/2
  b/1(b) -> Product3/2
  Add1/1 -> Sqrt/1
  Product3/1 -> Abs/1
  w/1 -> Abs1/1
  Constant/1 -> Add1/2
  Divide/1 -> Product2/2, Product2/1
  Iddej/1 -> Divide/1
  Sqrt/1 -> Product3/1

== system Model_IPS7/Regulacija3/Regulacija navora/Limita q toka/tokovna ==
  Id : Inport
  Abs : Abs
  Constant : Constant  Value=Ismax^2
  Gain2 : Gain  Gain=-1
  Product1 : Product
  Saturation : Saturate  UpperLimit=Ismax^2  LowerLimit=0  ZeroCross=off
  Sqrt : Sqrt  SaturateOnIntegerOverflow=on
  Subtract : Sum  Inputs=+-
  high : Outport
  low : Outport  Port=2
  wires:
  Subtract/1 -> Saturation/1
  Product1/1 -> Subtract/2
  Constant/1 -> Subtract/1
  Gain2/1 -> low/1
  Id/1 -> Product1/1, Product1/2
  Sqrt/1 -> Gain2/1, high/1
  Saturation/1 -> Abs/1
  Abs/1 -> Sqrt/1

== system Model_IPS7/Regulacija3/Transformacije/Clarke/ABC_ab1 ==
  A : Inport
  B : Inport  Port=2
  C : Inport  Port=3
  Gain1 : Gain  Gain=2
  Gain2 : Gain
  Gain24 : Gain  Gain=sqrt(3)/3
  Sum11 : Sum
  Terminator : Terminator
  alfa : Outport
  beta : Outport  Port=2
  wires:
  A/1 -> Gain2/1, Sum11/1
  Sum11/1 -> Gain24/1
  Gain2/1 -> alfa/1
  Gain24/1 -> beta/1
  B/1 -> Gain1/1
  Gain1/1 -> Sum11/2
  C/1 -> Terminator/1

== system Model_IPS7/Regulacija3/Transformacije/Inverzni Clarke/ab_ABC ==
  alfa : Inport
  beta : Inport  Port=2
  Gain1 : Gain
  Gain2 : Gain  Gain=-0.5
  Gain25 : Gain  Gain=sqrt(3)/2
  Gain3 : Gain  Gain=sqrt(3)/2
  Gain4 : Gain  Gain=0.5
  Sum10 : Sum
  Sum11 : Sum  Inputs=--
  A : Outport
  B : Outport  Port=2
  C : Outport  Port=3
  wires:
  Sum11/1 -> C/1
  Sum10/1 -> B/1
  Gain1/1 -> A/1
  alfa/1 -> Gain4/1, Gain2/1, Gain1/1
  Gain2/1 -> Sum10/1
  Gain25/1 -> Sum10/2
  Gain4/1 -> Sum11/1
  beta/1 -> Gain3/1, Gain25/1
  Gain3/1 -> Sum11/2

== system Model_IPS7/Regulacija1/Regulacija navora/Limita q toka/napetostna limita/a ==
  w : Inport
  Add3 : Sum
  Constant1 : Constant  Value=Udc/Ls
  Constant2 : Constant  Value=0.001
  Divide : Product  Inputs=*/
  a : Outport
  wires:
  Constant1/1 -> Divide/1
  Constant2/1 -> Add3/2
  Add3/1 -> Divide/2
  w/1 -> Add3/1
  Divide/1 -> a/1

== system Model_IPS7/Regulacija1/Regulacija navora/Limita q toka/napetostna limita/b ==
  w : Inport
  Add4 : Sum
  Constant3 : Constant  Value=Udc/Lst
  Constant4 : Constant  Value=0.001
  Divide1 : Product  Inputs=*/
  b : Outport
  wires:
  Divide1/1 -> b/1
  w/1 -> Add4/1
  Add4/1 -> Divide1/2
  Constant3/1 -> Divide1/1
  Constant4/1 -> Add4/2

== system Model_IPS7/Regulacija2/Regulacija navora/Limita q toka/napetostna limita/a ==
  w : Inport
  Add3 : Sum
  Constant1 : Constant  Value=Udc/Ls
  Constant2 : Constant  Value=0.001
  Divide : Product  Inputs=*/
  a : Outport
  wires:
  Constant1/1 -> Divide/1
  Constant2/1 -> Add3/2
  Add3/1 -> Divide/2
  w/1 -> Add3/1
  Divide/1 -> a/1

== system Model_IPS7/Regulacija2/Regulacija navora/Limita q toka/napetostna limita/b ==
  w : Inport
  Add4 : Sum
  Constant3 : Constant  Value=Udc/Lst
  Constant4 : Constant  Value=0.001
  Divide1 : Product  Inputs=*/
  b : Outport
  wires:
  Divide1/1 -> b/1
  w/1 -> Add4/1
  Add4/1 -> Divide1/2
  Constant3/1 -> Divide1/1
  Constant4/1 -> Add4/2

== system Model_IPS7/Regulacija3/Regulacija navora/Limita q toka/napetostna limita/a ==
  w : Inport
  Add3 : Sum
  Constant1 : Constant  Value=Udc/Ls
  Constant2 : Constant  Value=0.001
  Divide : Product  Inputs=*/
  a : Outport
  wires:
  Divide/1 -> a/1
  w/1 -> Add3/1
  Add3/1 -> Divide/2
  Constant2/1 -> Add3/2
  Constant1/1 -> Divide/1

== system Model_IPS7/Regulacija3/Regulacija navora/Limita q toka/napetostna limita/b ==
  w : Inport
  Add4 : Sum
  Constant3 : Constant  Value=Udc/Lst
  Constant4 : Constant  Value=0.001
  Divide1 : Product  Inputs=*/
  b : Outport
  wires:
  Constant4/1 -> Add4/2
  Constant3/1 -> Divide1/1
  Add4/1 -> Divide1/2
  w/1 -> Add4/1
  Divide1/1 -> b/1
